simulink model "uut_sdbe_pipeline"  (R2012b)
settings: Solver=ode45  StartTime=0.0  StopTime=sim_time  RelTol=1e-3
libraries: xbsIndex_r4 x1893, casper_library_misc x7, casper_library_delays x6, xps_library x1, r2dbe_vdif_lib x1
(part 1 of 15)
settings Model: Creator=lvertats  LastModifiedBy=lvertats

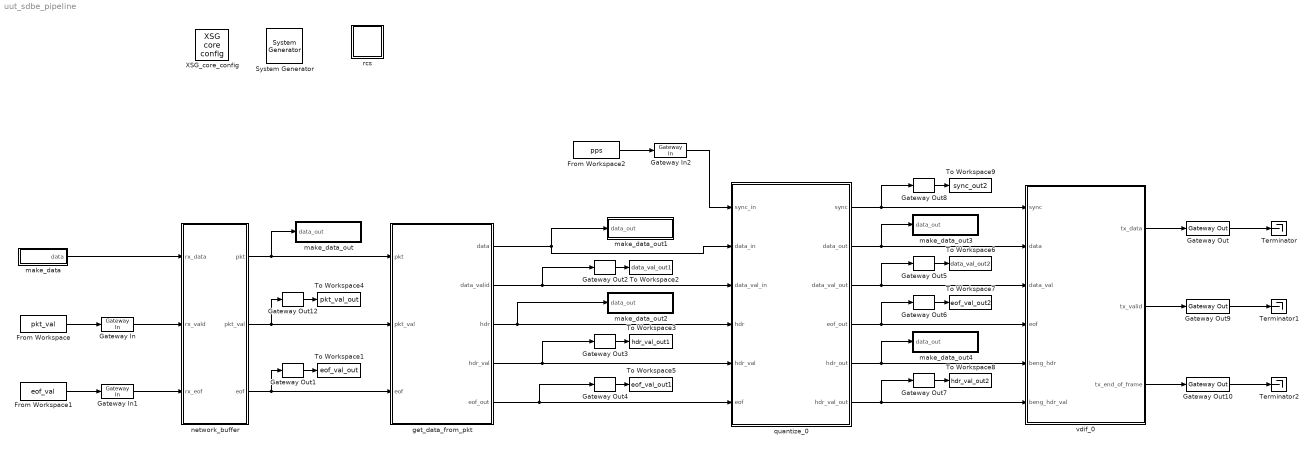
== system uut_sdbe_pipeline ==
  " System Generator" : xbsIndex_r4/ System Generator  Tag=genX  xilinxfamily=virtex6  part=xc6vsx475t  speed=-1  package=ff1759  synthesis_tool=XST  clock_wrapper=Clock Enables  directory=./sdbe_8_11/sysgen  proj_type=Project Navigator  Synth_file=XST Defaults  Impl_file=ISE Defaults  testbench=off  simulink_period=1  sysclk_period=4.8077  dcm_input_clock_period=100  incr_netlist=off  trim_vbits=Everywhere in SubSystem  dbl_ovrd=According to Block Masks  core_generation=According to Block Masks  run_coregen=off  deprecated_control=off  eval_field=0  block_type=sysgen
  From Workspace : FromWorkspace  VariableName=pkt_val  SampleTime=1  Interpolate=off  OutputAfterFinalValue=Setting to zero
  From Workspace1 : FromWorkspace  VariableName=eof_val  SampleTime=1  Interpolate=off  OutputAfterFinalValue=Setting to zero
  From Workspace2 : FromWorkspace  VariableName=pps  SampleTime=1  Interpolate=off  OutputAfterFinalValue=Setting to zero
  Gateway In : xbsIndex_r4/Gateway In  gui_display_data_type=Boolean  arith_type=Boolean  n_bits=16  bin_pt=14  preci_type=Single  exp_width=8  frac_width=24  quantization="Round  (unbiased: +/- Inf)"  overflow=Saturate  period=1  dbl_ovrd=off  timing_constraint=None  locs_specified=off  LOCs={}  UseAsADC=off  ADCChannel='1'  inherit_from_input=off  hdl_port=on  block_type=gatewayin
  Gateway In1 : xbsIndex_r4/Gateway In  gui_display_data_type=Boolean  arith_type=Boolean  n_bits=16  bin_pt=14  preci_type=Single  exp_width=8  frac_width=24  quantization="Round  (unbiased: +/- Inf)"  overflow=Saturate  period=1  dbl_ovrd=off  timing_constraint=None  locs_specified=off  LOCs={}  UseAsADC=off  ADCChannel='1'  inherit_from_input=off  hdl_port=on  block_type=gatewayin
  Gateway In2 : xbsIndex_r4/Gateway In  gui_display_data_type=Boolean  arith_type=Boolean  n_bits=16  bin_pt=14  preci_type=Single  exp_width=8  frac_width=24  quantization="Round  (unbiased: +/- Inf)"  overflow=Saturate  period=1  dbl_ovrd=off  timing_constraint=None  locs_specified=off  LOCs={}  UseAsADC=off  ADCChannel='1'  inherit_from_input=off  hdl_port=on  block_type=gatewayin
  Gateway Out{,1..10,12} (12 alike) : xbsIndex_r4/Gateway Out  inherit_from_input=off  hdl_port=on  timing_constraint=None  locs_specified=off  LOCs={}  UseAsDAC=off  DACChannel='1'  block_type=gatewayout
  Terminator : Terminator
  Terminator1 : Terminator
  Terminator2 : Terminator
  To Workspace1 : ToWorkspace  VariableName=eof_val_out  SampleTime=-1  SaveFormat=Timeseries
  To Workspace2 : ToWorkspace  VariableName=data_val_out1  SampleTime=-1  SaveFormat=Timeseries
  To Workspace3 : ToWorkspace  VariableName=hdr_val_out1  SampleTime=-1  SaveFormat=Timeseries
  To Workspace4 : ToWorkspace  VariableName=pkt_val_out  SampleTime=-1  SaveFormat=Timeseries
  To Workspace5 : ToWorkspace  VariableName=eof_val_out1  SampleTime=-1  SaveFormat=Timeseries
  To Workspace6 : ToWorkspace  VariableName=data_val_out2  SampleTime=-1  SaveFormat=Timeseries
  To Workspace7 : ToWorkspace  VariableName=eof_val_out2  SampleTime=-1  SaveFormat=Timeseries
  To Workspace8 : ToWorkspace  VariableName=hdr_val_out2  SampleTime=-1  SaveFormat=Timeseries
  To Workspace9 : ToWorkspace  VariableName=sync_out2  SampleTime=-1  SaveFormat=Timeseries
  XSG_core_config : xps_library/XSG core config  Tag=xps:xsg  hw_sys=ROACH2:sx475t  clk_src=adc0_clk  ROACH_clk_src=sys_clk  ROACH2_clk_src=adc0_clk  MKDIG_clk_src=sys_clk  clk_rate=3328/16  sample_period=1  synthesis_tool=XST
  get_data_from_pkt : Subsystem
  make_data : Subsystem
  make_data_out : Subsystem
  make_data_out1 : Subsystem
  make_data_out2 : Subsystem
  make_data_out3 : Subsystem
  make_data_out4 : Subsystem
  network_buffer : Subsystem
  quantize_0 : Subsystem  mask(r2dbe_quantize){mult_delay=3, add_delay=2, convert_delay=1, pipeline_delay=1, io_delay=3}
      mask prompts: mult_delay "Multiplier latency:"; add_delay "Adder latency:"; convert_delay "Convert latency:"; pipeline_delay "Output pipeline delay:"; io_delay "I/O delay:"
      mask help: Sub-system for quantization parameters of the R2DBE.
  rcs : Subsystem  AncestorBlock=casper_library_misc/rcs  mask(rcs){app_src=timestamp, lib_src=timestamp, user_val=0}
      mask prompts: app_src "Application revision info to capture"; lib_src "CASPER libraries revision info to capture"; user_val "User specified value"
      mask help:
      | Embeds revision control information for the user design and libraries.
      | On failure to locate specified revision information, falls back to
      | timestamps (current time for libraries).
      | A user specified value is also stored.
      mask init:
      | rcs_init(gcb, ...
      |     'app_src', app_src, ...
      |     'lib_src', lib_src);
      mask TypeOptions app_src: timestamp | git | svn
      mask TypeOptions lib_src: timestamp | git | svn
  vdif_0 : Subsystem  mask(r2dbe_vdif){}
      mask help: Sub-system for VDIF parameters of the R2DBE.
  wires:
  From Workspace1/1 -> Gateway In1/1
  From Workspace/1 -> Gateway In/1
  Gateway In/1 -> network_buffer/2(rx_vald)
  Gateway In1/1 -> network_buffer/3(rx_eof)
  make_data/1(data) -> network_buffer/1(rx_data)
  network_buffer/1(pkt) -> make_data_out/1(data_out), get_data_from_pkt/1(pkt)
  Gateway Out12/1 -> To Workspace4/1
  network_buffer/2(pkt_val) -> Gateway Out12/1, get_data_from_pkt/2(pkt_val)
  Gateway Out1/1 -> To Workspace1/1
  network_buffer/3(eof) -> Gateway Out1/1, get_data_from_pkt/3(eof)
  get_data_from_pkt/1(data) -> quantize_0/2(data_in), make_data_out1/1(data_out)
  Gateway Out2/1 -> To Workspace2/1
  get_data_from_pkt/2(data_valid) -> Gateway Out2/1, quantize_0/3(data_val_in)
  Gateway Out3/1 -> To Workspace3/1
  get_data_from_pkt/4(hdr_val) -> quantize_0/5(hdr_val), Gateway Out3/1
  get_data_from_pkt/3(hdr) -> quantize_0/4(hdr), make_data_out2/1(data_out)
  Gateway Out4/1 -> To Workspace5/1
  get_data_from_pkt/5(eof_out) -> quantize_0/6(eof), Gateway Out4/1
  From Workspace2/1 -> Gateway In2/1
  Gateway In2/1 -> quantize_0/1(sync_in)
  quantize_0/2(data_out) -> vdif_0/2(data), make_data_out3/1(data_out)
  Gateway Out5/1 -> To Workspace6/1
  quantize_0/3(data_val_out) -> vdif_0/3(data_val), Gateway Out5/1
  quantize_0/5(hdr_out) -> vdif_0/5(beng_hdr), make_data_out4/1(data_out)
  Gateway Out6/1 -> To Workspace7/1
  quantize_0/4(eof_out) -> vdif_0/4(eof), Gateway Out6/1
  Gateway Out7/1 -> To Workspace8/1
  quantize_0/6(hdr_val_out) -> vdif_0/6(beng_hdr_val), Gateway Out7/1
  Gateway Out8/1 -> To Workspace9/1
  quantize_0/1(sync) -> Gateway Out8/1, vdif_0/1(sync)
  Gateway Out/1 -> Terminator/1
  vdif_0/1(tx_data) -> Gateway Out/1
  Gateway Out9/1 -> Terminator1/1
  vdif_0/2(tx_valid) -> Gateway Out9/1
  Gateway Out10/1 -> Terminator2/1
  vdif_0/3(tx_end_of_frame) -> Gateway Out10/1

== system uut_sdbe_pipeline/get_data_from_pkt ==
  note: SHOULD BE AN AND HERE ON EOF AND DATA VAL GOING OUT EOF
  note: can pass all through, but turn valid off for first
  pkt : Inport
  pkt_val : Inport  Port=2
  eof : Inport  Port=3
  Constant : Constant  Value=0
  Counter : xbsIndex_r4/Counter  cnt_type=Free Running  cnt_to=Inf  operation=Up  start_count=0  cnt_by_val=1  arith_type=Unsigned  n_bits=32  bin_pt=0  load_pin=off  rst=on  en=on  explicit_period=on  period=1  dbl_ovrd=off  use_behavioral_HDL=off  implementation=Fabric  block_type=counter
  Delay2 : xbsIndex_r4/Delay  rst=off  infoeditControl=Selection of Reset will increase slice count due to use of real FFs and instead of SRLs  en=off  latency=1  dbl_ovrd=off  reg_retiming=off  block_type=delay
  Delay3 : xbsIndex_r4/Delay  rst=off  infoeditControl=Selection of Reset will increase slice count due to use of real FFs and instead of SRLs  en=off  latency=1  dbl_ovrd=off  reg_retiming=off  block_type=delay
  Slice : xbsIndex_r4/Slice  nbits=1  boolean_output=on  mode=Upper Bit Location + Width  bit1=0  base1=MSB of Input  bit0=0  base0=LSB of Input  dbl_ovrd=off  block_type=slice
  Terminator : Terminator
  gen_valids1 : Subsystem
      mask help: latency 1
  npkts : Subsystem  Tag=xps:sw_reg  AncestorBlock=xps_library/software register  mask(swreg){mode=one value, io_dir=To Processor, io_delay=0, sample_period=1, names=reg, bitwidths=32, arith_types=0, bin_pts=0, sim_port=on, show_format=off}
      mask prompts: io_dir "I/O direction"; io_delay "I/O delay"; sample_period "Sample period"; names "Name:"; bitwidths "Bitwidth:"; arith_types "Type (ufix=0, fix=1, bool=2):"; bin_pts "Binary pt:"; sim_port "Provide sim input/output?"; show_format "Print format string?"
      mask init:
      | swreg_init(gcb)
      settings: AttributesFormatString=1output
      mask TypeOptions mode: one value | fields of equal size | fields of arbitrary size
      mask Callback mode: swreg_cb(gcb);
      mask TypeOptions io_dir: To Processor | From Processor
      mask Callback io_dir:
      | mask_enables = get_param(gcb, 'MaskEnables');
      | mask_names = get_param(gcb, 'MaskNames');
      | if strcmp(get_param(gcb, 'io_dir'), 'To Processor'),
      |     mask_enables{ismember(mask_names, 'sample_period')} = 'off';
      | else
      |     mask_enables{ismember(mask_names, 'sample_period')} = 'on';
      | end
      | set_param(gcb, 'MaskEnables', mask_enables);
      mask Callback bitwidths:
      | swreg_maskcheck(gcb);
      | % blk = gcb;
      | % mode = get_param(blk, 'mode');
      | % current_widths = eval(get_param(blk, 'bitwidths'));
      | % if (strcmp(mode, 'one value') || strcmp(mode, 'fields of equal size')) && (length(current_widths) > 1),
      | %     error('Only one width may be specified for this mode.');
      | % elseif strcmp(mode, 'fields of arbitrary size')
      | %     current_names = textscan(strtrim(strrep(strrep(get_param(blk, 'names'), ']', ''), '[', '')), '%s');
      | %     current_names = current_names{1};
      | %     numios = length(current_names);
      | %     if length(current_widths) ~= numios,
      | %         error('%d field names specified, but %d widths?', numios, length(current_widths));
      | %     end
      | % end
      | % total_width = 0;
      | % for ctr = 1 : length(current_widths),
      | %     total_width = total_width + current_widths(ctr);
      | % end
      | % if total_width > 32,
      | %     error('Total width must be 32 or less, set to %d.', total_width);
      | % end
      mask Callback arith_types:
      | [numios, ~, ~, ~, current_types] = swreg_maskcheck(gcb);
      | % blk = gcb;
      | % mode = get_param(blk, 'mode');
      | % current_types = eval(get_param(blk, 'arith_types'));
      | % numios = length(current_types);
      | % if (strcmp(mode, 'one value') || strcmp(mode, 'fields of equal size')) && (length(current_types) > 1),
      | %     error('Only one type may be specified for this mode.');
      | % elseif strcmp(mode, 'fields of arbitrary size')
      | %     current_names = textscan(strtrim(strrep(strrep(get_param(blk, 'names'), ']', ''), '[', '')), '%s');
      | %     current_names = current_names{1};
      | %     numios = length(current_names);
      | %     if length(current_types) ~= numios,
      | %         error('%d field names specified, but %d types?', numios, length(current_types));
      | %     end
      | % end
      | problem = 0;
      | for ctr = 1 : numios,
      |     t = current_types(ctr);
      |     if (t < 0) || (t > 2),
      |         problem = t;
      |         ctr = numios + 1;
      |     end
      | end
      | if problem ~= 0,
      |     error('Type cannot be %i, must be 0, 1 or 2.', problem);
      | end
      mask Callback bin_pts:
      | swreg_maskcheck(gcb);
      | % blk = gcb;
      | % mode = get_param(blk, 'mode');
      | % current_bins = eval(get_param(blk, 'bin_pts'));
      | % if (strcmp(mode, 'one value') || strcmp(mode, 'fields of equal size')) && (length(current_bins) > 1),
      | %     error('Only one binary pt may be specified for this mode.');
      | % elseif strcmp(mode, 'fields of arbitrary size')
      | %     current_names = textscan(strtrim(strrep(strrep(get_param(blk, 'names'), ']', ''), '[', '')), '%s');
      | %     current_names = current_names{1};
      | %     numios = length(current_names);
      | %     if length(current_bins) ~= numios,
      | %         error('%d field names specified, but %d binary pts?', numios, length(current_bins));
      | %     end
      | % end
  rst : Subsystem  Tag=xps:sw_reg  AncestorBlock=xps_library/software register  mask(swreg){mode=one value, io_dir=From Processor, io_delay=0, sample_period=1, names=reg, bitwidths=32, arith_types=0, bin_pts=0, sim_port=on, show_format=off}
      mask prompts: io_dir "I/O direction"; io_delay "I/O delay"; sample_period "Sample period"; names "Name:"; bitwidths "Bitwidth:"; arith_types "Type (ufix=0, fix=1, bool=2):"; bin_pts "Binary pt:"; sim_port "Provide sim input/output?"; show_format "Print format string?"
      mask init:
      | swreg_init(gcb)
      settings: AttributesFormatString=1input
      mask TypeOptions mode: one value | fields of equal size | fields of arbitrary size
      mask Callback mode: swreg_cb(gcb);
      mask TypeOptions io_dir: To Processor | From Processor
      mask Callback io_dir:
      | mask_enables = get_param(gcb, 'MaskEnables');
      | mask_names = get_param(gcb, 'MaskNames');
      | if strcmp(get_param(gcb, 'io_dir'), 'To Processor'),
      |     mask_enables{ismember(mask_names, 'sample_period')} = 'off';
      | else
      |     mask_enables{ismember(mask_names, 'sample_period')} = 'on';
      | end
      | set_param(gcb, 'MaskEnables', mask_enables);
      mask Callback bitwidths:
      | swreg_maskcheck(gcb);
      | % blk = gcb;
      | % mode = get_param(blk, 'mode');
      | % current_widths = eval(get_param(blk, 'bitwidths'));
      | % if (strcmp(mode, 'one value') || strcmp(mode, 'fields of equal size')) && (length(current_widths) > 1),
      | %     error('Only one width may be specified for this mode.');
      | % elseif strcmp(mode, 'fields of arbitrary size')
      | %     current_names = textscan(strtrim(strrep(strrep(get_param(blk, 'names'), ']', ''), '[', '')), '%s');
      | %     current_names = current_names{1};
      | %     numios = length(current_names);
      | %     if length(current_widths) ~= numios,
      | %         error('%d field names specified, but %d widths?', numios, length(current_widths));
      | %     end
      | % end
      | % total_width = 0;
      | % for ctr = 1 : length(current_widths),
      | %     total_width = total_width + current_widths(ctr);
      | % end
      | % if total_width > 32,
      | %     error('Total width must be 32 or less, set to %d.', total_width);
      | % end
      mask Callback arith_types:
      | [numios, ~, ~, ~, current_types] = swreg_maskcheck(gcb);
      | % blk = gcb;
      | % mode = get_param(blk, 'mode');
      | % current_types = eval(get_param(blk, 'arith_types'));
      | % numios = length(current_types);
      | % if (strcmp(mode, 'one value') || strcmp(mode, 'fields of equal size')) && (length(current_types) > 1),
      | %     error('Only one type may be specified for this mode.');
      | % elseif strcmp(mode, 'fields of arbitrary size')
      | %     current_names = textscan(strtrim(strrep(strrep(get_param(blk, 'names'), ']', ''), '[', '')), '%s');
      | %     current_names = current_names{1};
      | %     numios = length(current_names);
      | %     if length(current_types) ~= numios,
      | %         error('%d field names specified, but %d types?', numios, length(current_types));
      | %     end
      | % end
      | problem = 0;
      | for ctr = 1 : numios,
      |     t = current_types(ctr);
      |     if (t < 0) || (t > 2),
      |         problem = t;
      |         ctr = numios + 1;
      |     end
      | end
      | if problem ~= 0,
      |     error('Type cannot be %i, must be 0, 1 or 2.', problem);
      | end
      mask Callback bin_pts:
      | swreg_maskcheck(gcb);
      | % blk = gcb;
      | % mode = get_param(blk, 'mode');
      | % current_bins = eval(get_param(blk, 'bin_pts'));
      | % if (strcmp(mode, 'one value') || strcmp(mode, 'fields of equal size')) && (length(current_bins) > 1),
      | %     error('Only one binary pt may be specified for this mode.');
      | % elseif strcmp(mode, 'fields of arbitrary size')
      | %     current_names = textscan(strtrim(strrep(strrep(get_param(blk, 'names'), ']', ''), '[', '')), '%s');
      | %     current_names = current_names{1};
      | %     numios = length(current_names);
      | %     if length(current_bins) ~= numios,
      | %         error('%d field names specified, but %d binary pts?', numios, length(current_bins));
      | %     end
      | % end
  rx_output : Subsystem
  rx_output1 : Subsystem
  scope : Subsystem
  data : Outport
  data_valid : Outport  Port=2
  hdr : Outport  Port=3
  hdr_val : Outport  Port=4
  eof_out : Outport  Port=5
  wires:
  pkt/1 -> Delay2/1
  Delay2/1 -> [data], data/1, [hdr], hdr/1
  Delay3/1 -> [eof], eof_out/1
  eof/1 -> gen_valids1/2(eof), Delay3/1
  npkts/1(sim_out) -> Terminator/1
  Counter/1 -> npkts/1(out_reg)
  rst/1(in_reg) -> Slice/1
  Constant/1 -> rst/1(sim_1)
  Slice/1 -> Counter/1
  pkt_val/1 -> gen_valids1/1(pkt_val)
  gen_valids1/1(hdr_val) -> [hdr_val], hdr_val/1
  gen_valids1/2(data_val) -> [data_val], data_valid/1
  [eof] -> Counter/2
  [data_val] -> rx_output/2(val)
  [eof] -> rx_output/3(eof)
  [hdr_val] -> rx_output/1(sig)
  [data] -> rx_output1/3(data)
  [hdr] -> rx_output1/1(hdr)
  [hdr_val] -> rx_output1/2(hdr_val)
  [data_val] -> rx_output1/4(data_val)
  [data_val] -> scope/2(valid)
  [data] -> scope/1(data)

== system uut_sdbe_pipeline/make_data ==
  Concat : xbsIndex_r4/Concat  num_inputs=2  dbl_ovrd=off  block_type=concat
  From Workspace1 : FromWorkspace  VariableName=data_top  Interpolate=off  OutputAfterFinalValue=Cyclic repetition
  From Workspace2 : FromWorkspace  VariableName=data_bott  Interpolate=off  OutputAfterFinalValue=Cyclic repetition
  Gateway In1 : xbsIndex_r4/Gateway In  gui_display_data_type=Fixed-point  arith_type=Unsigned  n_bits=32  bin_pt=0  preci_type=Single  exp_width=8  frac_width=24  quantization="Round  (unbiased: +/- Inf)"  overflow=Saturate  period=1  dbl_ovrd=off  timing_constraint=None  locs_specified=off  LOCs={}  UseAsADC=off  ADCChannel='1'  inherit_from_input=off  hdl_port=on  block_type=gatewayin
  Gateway In15 : xbsIndex_r4/Gateway In  gui_display_data_type=Fixed-point  arith_type=Unsigned  n_bits=32  bin_pt=0  preci_type=Single  exp_width=8  frac_width=24  quantization="Round  (unbiased: +/- Inf)"  overflow=Saturate  period=1  dbl_ovrd=off  timing_constraint=None  locs_specified=off  LOCs={}  UseAsADC=off  ADCChannel='1'  inherit_from_input=off  hdl_port=on  block_type=gatewayin
  data : Outport
  wires:
  Concat/1 -> data/1
  Gateway In15/1 -> Concat/1
  From Workspace1/1 -> Gateway In15/1
  Gateway In1/1 -> Concat/2
  From Workspace2/1 -> Gateway In1/1

== system uut_sdbe_pipeline/make_data_out ==
  data_out : Inport
  Gateway Out6 : xbsIndex_r4/Gateway Out  inherit_from_input=off  hdl_port=on  timing_constraint=None  locs_specified=off  LOCs={}  UseAsDAC=off  DACChannel='1'  block_type=gatewayout
  Gateway Out7 : xbsIndex_r4/Gateway Out  inherit_from_input=off  hdl_port=on  timing_constraint=None  locs_specified=off  LOCs={}  UseAsDAC=off  DACChannel='1'  block_type=gatewayout
  To Workspace13 : ToWorkspace  VariableName=data_top_out  SampleTime=-1  SaveFormat=Timeseries
  To Workspace9 : ToWorkspace  VariableName=data_bott_out  SampleTime=-1  SaveFormat=Timeseries
  bus_expand : Subsystem  AncestorBlock=casper_library_flow_control/bus_expand  mask(bus_expand){mode=divisions of equal size, outputNum=2, outputWidth=32, outputBinaryPt=0, outputArithmeticType=0, show_format=off, outputToWorkspace=off, variablePrefix=out, outputToModelAsWell=on}
      mask prompts: outputNum "Number of outputs:"; outputWidth "Output width:"; outputBinaryPt "Output binary point position:"; outputArithmeticType "Output arithmetic type (ufix=0, fix=1, bool=2):"; show_format "Print format string?"; outputToWorkspace "Output to workspace?"; variablePrefix "Variable name prefix:"; outputToModelAsWell "Output to model as well?"
      mask help:
      | Expands a 'bus' made using a bus_create or Xilinx
      | concat block.
      | The input will be divided into the specified number
      | of outputs with the specified arithmetic types.
      | Divisions are made from most significant bit.
      mask init:
      | bus_expand_init(gcb,...
      |     'mode', mode, ...
      |     'outputNum', outputNum, ...
      |     'outputWidth', outputWidth, ...
      |     'outputBinaryPt', outputBinaryPt, ...
      |     'outputArithmeticType', outputArithmeticType, ...
      |     'show_format', show_format, ...
      |     'outputToWorkspace', outputToWorkspace, ...
      |     'variablePrefix', variablePrefix, ...
      |     'outputToModelAsWell', outputToModelAsWell);
      settings: AttributesFormatString=2 outputs
      mask TypeOptions mode: divisions of equal size | divisions of arbitrary size
      mask Callback mode: bus_expand_callback();
      mask Callback outputWidth: bus_expand_callback();
      mask Callback outputToWorkspace: bus_expand_callback();
  wires:
  data_out/1 -> bus_expand/1(bus_in)
  Gateway Out7/1 -> To Workspace9/1
  Gateway Out6/1 -> To Workspace13/1
  bus_expand/1(msb_out2) -> Gateway Out6/1
  bus_expand/2(lsb_out1) -> Gateway Out7/1

== system uut_sdbe_pipeline/make_data_out1 ==
  data_out : Inport
  Gateway Out6 : xbsIndex_r4/Gateway Out  inherit_from_input=off  hdl_port=on  timing_constraint=None  locs_specified=off  LOCs={}  UseAsDAC=off  DACChannel='1'  block_type=gatewayout
  Gateway Out7 : xbsIndex_r4/Gateway Out  inherit_from_input=off  hdl_port=on  timing_constraint=None  locs_specified=off  LOCs={}  UseAsDAC=off  DACChannel='1'  block_type=gatewayout
  To Workspace13 : ToWorkspace  VariableName=data_top_out1  SampleTime=-1  SaveFormat=Timeseries
  To Workspace9 : ToWorkspace  VariableName=data_bott_out1  SampleTime=-1  SaveFormat=Timeseries
  bus_expand : Subsystem  AncestorBlock=casper_library_flow_control/bus_expand  mask(bus_expand){mode=divisions of equal size, outputNum=2, outputWidth=32, outputBinaryPt=0, outputArithmeticType=0, show_format=off, outputToWorkspace=off, variablePrefix=out, outputToModelAsWell=on}
      mask prompts: outputNum "Number of outputs:"; outputWidth "Output width:"; outputBinaryPt "Output binary point position:"; outputArithmeticType "Output arithmetic type (ufix=0, fix=1, bool=2):"; show_format "Print format string?"; outputToWorkspace "Output to workspace?"; variablePrefix "Variable name prefix:"; outputToModelAsWell "Output to model as well?"
      mask help:
      | Expands a 'bus' made using a bus_create or Xilinx
      | concat block.
      | The input will be divided into the specified number
      | of outputs with the specified arithmetic types.
      | Divisions are made from most significant bit.
      mask init: same as uut_sdbe_pipeline/make_data_out/bus_expand
      settings: AttributesFormatString=2 outputs
      mask TypeOptions mode: divisions of equal size | divisions of arbitrary size
      mask Callback mode: bus_expand_callback();
      mask Callback outputWidth: bus_expand_callback();
      mask Callback outputToWorkspace: bus_expand_callback();
  wires:
  bus_expand/2(lsb_out1) -> Gateway Out7/1
  bus_expand/1(msb_out2) -> Gateway Out6/1
  Gateway Out6/1 -> To Workspace13/1
  Gateway Out7/1 -> To Workspace9/1
  data_out/1 -> bus_expand/1(bus_in)

== system uut_sdbe_pipeline/make_data_out2 ==
  data_out : Inport
  Gateway Out6 : xbsIndex_r4/Gateway Out  inherit_from_input=off  hdl_port=on  timing_constraint=None  locs_specified=off  LOCs={}  UseAsDAC=off  DACChannel='1'  block_type=gatewayout
  Gateway Out7 : xbsIndex_r4/Gateway Out  inherit_from_input=off  hdl_port=on  timing_constraint=None  locs_specified=off  LOCs={}  UseAsDAC=off  DACChannel='1'  block_type=gatewayout
  To Workspace13 : ToWorkspace  VariableName=hdr_top_out1  SampleTime=-1  SaveFormat=Timeseries
  To Workspace9 : ToWorkspace  VariableName=hdr_bott_out1  SampleTime=-1  SaveFormat=Timeseries
  bus_expand : Subsystem  AncestorBlock=casper_library_flow_control/bus_expand  mask(bus_expand){mode=divisions of equal size, outputNum=2, outputWidth=32, outputBinaryPt=0, outputArithmeticType=0, show_format=off, outputToWorkspace=off, variablePrefix=out, outputToModelAsWell=on}
      mask prompts: outputNum "Number of outputs:"; outputWidth "Output width:"; outputBinaryPt "Output binary point position:"; outputArithmeticType "Output arithmetic type (ufix=0, fix=1, bool=2):"; show_format "Print format string?"; outputToWorkspace "Output to workspace?"; variablePrefix "Variable name prefix:"; outputToModelAsWell "Output to model as well?"
      mask help:
      | Expands a 'bus' made using a bus_create or Xilinx
      | concat block.
      | The input will be divided into the specified number
      | of outputs with the specified arithmetic types.
      | Divisions are made from most significant bit.
      mask init: same as uut_sdbe_pipeline/make_data_out/bus_expand
      settings: AttributesFormatString=2 outputs
      mask TypeOptions mode: divisions of equal size | divisions of arbitrary size
      mask Callback mode: bus_expand_callback();
      mask Callback outputWidth: bus_expand_callback();
      mask Callback outputToWorkspace: bus_expand_callback();
  wires:
  data_out/1 -> bus_expand/1(bus_in)
  Gateway Out7/1 -> To Workspace9/1
  Gateway Out6/1 -> To Workspace13/1
  bus_expand/1(msb_out2) -> Gateway Out6/1
  bus_expand/2(lsb_out1) -> Gateway Out7/1

== system uut_sdbe_pipeline/make_data_out3 ==
  data_out : Inport
  Gateway Out6 : xbsIndex_r4/Gateway Out  inherit_from_input=off  hdl_port=on  timing_constraint=None  locs_specified=off  LOCs={}  UseAsDAC=off  DACChannel='1'  block_type=gatewayout
  Gateway Out7 : xbsIndex_r4/Gateway Out  inherit_from_input=off  hdl_port=on  timing_constraint=None  locs_specified=off  LOCs={}  UseAsDAC=off  DACChannel='1'  block_type=gatewayout
  To Workspace13 : ToWorkspace  VariableName=data_top_out2  SampleTime=-1  SaveFormat=Timeseries
  To Workspace9 : ToWorkspace  VariableName=data_bott_out2  SampleTime=-1  SaveFormat=Timeseries
  bus_expand : Subsystem  AncestorBlock=casper_library_flow_control/bus_expand  mask(bus_expand){mode=divisions of equal size, outputNum=2, outputWidth=16, outputBinaryPt=0, outputArithmeticType=0, show_format=off, outputToWorkspace=off, variablePrefix=out, outputToModelAsWell=on}
      mask prompts: outputNum "Number of outputs:"; outputWidth "Output width:"; outputBinaryPt "Output binary point position:"; outputArithmeticType "Output arithmetic type (ufix=0, fix=1, bool=2):"; show_format "Print format string?"; outputToWorkspace "Output to workspace?"; variablePrefix "Variable name prefix:"; outputToModelAsWell "Output to model as well?"
      mask help:
      | Expands a 'bus' made using a bus_create or Xilinx
      | concat block.
      | The input will be divided into the specified number
      | of outputs with the specified arithmetic types.
      | Divisions are made from most significant bit.
      mask init: same as uut_sdbe_pipeline/make_data_out/bus_expand
      settings: AttributesFormatString=2 outputs
      mask TypeOptions mode: divisions of equal size | divisions of arbitrary size
      mask Callback mode: bus_expand_callback();
      mask Callback outputWidth: bus_expand_callback();
      mask Callback outputToWorkspace: bus_expand_callback();
  wires:
  data_out/1 -> bus_expand/1(bus_in)
  Gateway Out7/1 -> To Workspace9/1
  Gateway Out6/1 -> To Workspace13/1
  bus_expand/1(msb_out2) -> Gateway Out6/1
  bus_expand/2(lsb_out1) -> Gateway Out7/1

== system uut_sdbe_pipeline/make_data_out4 ==
  data_out : Inport
  Gateway Out6 : xbsIndex_r4/Gateway Out  inherit_from_input=off  hdl_port=on  timing_constraint=None  locs_specified=off  LOCs={}  UseAsDAC=off  DACChannel='1'  block_type=gatewayout
  Gateway Out7 : xbsIndex_r4/Gateway Out  inherit_from_input=off  hdl_port=on  timing_constraint=None  locs_specified=off  LOCs={}  UseAsDAC=off  DACChannel='1'  block_type=gatewayout
  To Workspace13 : ToWorkspace  VariableName=hdr_top_out2  SampleTime=-1  SaveFormat=Timeseries
  To Workspace9 : ToWorkspace  VariableName=hdr_bott_out2  SampleTime=-1  SaveFormat=Timeseries
  bus_expand : Subsystem  AncestorBlock=casper_library_flow_control/bus_expand  mask(bus_expand){mode=divisions of equal size, outputNum=2, outputWidth=32, outputBinaryPt=0, outputArithmeticType=0, show_format=off, outputToWorkspace=off, variablePrefix=out, outputToModelAsWell=on}
      mask prompts: outputNum "Number of outputs:"; outputWidth "Output width:"; outputBinaryPt "Output binary point position:"; outputArithmeticType "Output arithmetic type (ufix=0, fix=1, bool=2):"; show_format "Print format string?"; outputToWorkspace "Output to workspace?"; variablePrefix "Variable name prefix:"; outputToModelAsWell "Output to model as well?"
      mask help:
      | Expands a 'bus' made using a bus_create or Xilinx
      | concat block.
      | The input will be divided into the specified number
      | of outputs with the specified arithmetic types.
      | Divisions are made from most significant bit.
      mask init: same as uut_sdbe_pipeline/make_data_out/bus_expand
      settings: AttributesFormatString=2 outputs
      mask TypeOptions mode: divisions of equal size | divisions of arbitrary size
      mask Callback mode: bus_expand_callback();
      mask Callback outputWidth: bus_expand_callback();
      mask Callback outputToWorkspace: bus_expand_callback();
  wires:
  bus_expand/2(lsb_out1) -> Gateway Out7/1
  bus_expand/1(msb_out2) -> Gateway Out6/1
  Gateway Out6/1 -> To Workspace13/1
  Gateway Out7/1 -> To Workspace9/1
  data_out/1 -> bus_expand/1(bus_in)
